simulink model "sim_Test"  (R2018a)
settings: Solver=FixedStepAuto  StartTime=0.0  StopTime=WIND(end,1)  FixedStep=0.01  RelTol=1e-3
values from neighbouring files (symbols this model uses):
  a = 0.015    [pwm_calib.mat]    (also in thr2pwm.mat)
  a1 = 3.041    [pwm_calib.mat]    (also in thr2pwm.mat)
  a2 = 1.679    [pwm_calib.mat]    (also in thr2pwm.mat)
  b = 1.686    [pwm_calib.mat]    (also in thr2pwm.mat)
  b1 = 0.1529    [pwm_calib.mat]    (also in thr2pwm.mat)
  b2 = 0.252    [pwm_calib.mat]    (also in thr2pwm.mat)
  c1 = -0.9269    [pwm_calib.mat]    (also in thr2pwm.mat)
  c2 = 1.268    [pwm_calib.mat]    (also in thr2pwm.mat)
settings Model: Creator=adiravishankara  LastModifiedBy=adiravishankara
settings DataIOCC: SaveFormat=Array

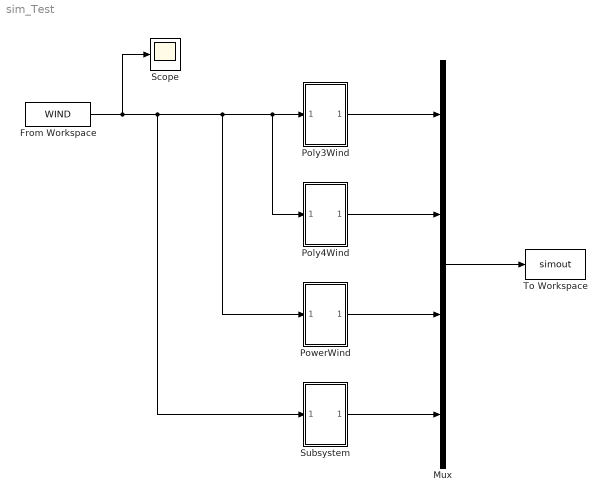
== system sim_Test ==
  From Workspace : FromWorkspace  VariableName=WIND
  Mux : Mux
  "Poly3Wind " : Subsystem
  "Poly4Wind " : Subsystem
  PowerWind : Subsystem
  Scope : Scope
  Subsystem : Subsystem
  To Workspace : ToWorkspace  VariableName=simout  SampleTime=-1
  wires:
  From Workspace/1 -> Scope/1, Subsystem/1(In1), PowerWind/1(In1), "Poly4Wind "/1(In1), "Poly3Wind "/1(In1)
  "Poly3Wind "/1(Out1) -> Mux/1
  "Poly4Wind "/1(Out1) -> Mux/2
  Subsystem/1(Out1) -> Mux/4
  PowerWind/1(Out1) -> Mux/3
  Mux/1 -> To Workspace/1

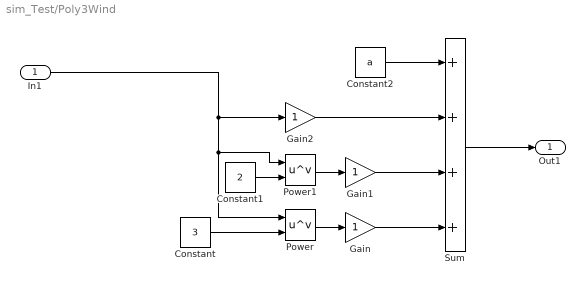
== system sim_Test/Poly3Wind  ==
  In1 : Inport
  Constant : Constant  Value=3
  Constant1 : Constant  Value=2
  Constant2 : Constant  Value=a
  Gain : Gain
  Gain1 : Gain
  Gain2 : Gain
  Power : Math  Operator=pow  SaturateOnIntegerOverflow=on
  Power1 : Math  Operator=pow  SaturateOnIntegerOverflow=on
  Sum : Sum  Inputs=++++
  Out1 : Outport
  wires:
  Constant2/1 -> Sum/1
  Constant1/1 -> Power1/2
  Gain2/1 -> Sum/2
  Sum/1 -> Out1/1
  Constant/1 -> Power/2
  Gain1/1 -> Sum/3
  In1/1 -> Gain2/1, Power1/1, Power/1
  Power1/1 -> Gain1/1
  Power/1 -> Gain/1
  Gain/1 -> Sum/4

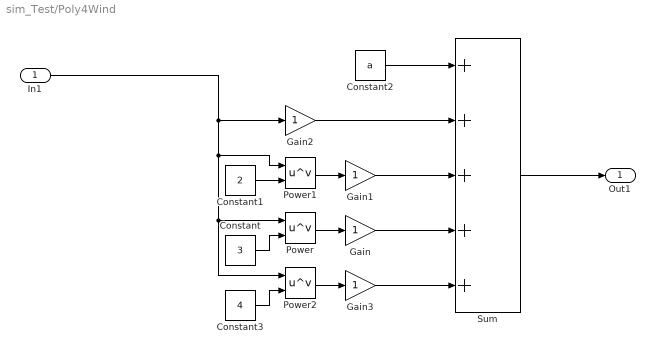
== system sim_Test/Poly4Wind  ==
  In1 : Inport
  Constant : Constant  Value=3
  Constant1 : Constant  Value=2
  Constant2 : Constant  Value=a
  Constant3 : Constant  Value=4
  Gain{,1..3} (4 alike) : Gain
  Power : Math  Operator=pow  SaturateOnIntegerOverflow=on
  Power1 : Math  Operator=pow  SaturateOnIntegerOverflow=on
  Power2 : Math  Operator=pow  SaturateOnIntegerOverflow=on
  Sum : Sum  Inputs=+++++
  Out1 : Outport
  wires:
  Gain/1 -> Sum/4
  Power/1 -> Gain/1
  Power1/1 -> Gain1/1
  In1/1 -> Power2/1, Power/1, Power1/1, Gain2/1
  Gain1/1 -> Sum/3
  Constant/1 -> Power/2
  Sum/1 -> Out1/1
  Gain2/1 -> Sum/2
  Constant1/1 -> Power1/2
  Constant2/1 -> Sum/1
  Constant3/1 -> Power2/2
  Power2/1 -> Gain3/1
  Gain3/1 -> Sum/5

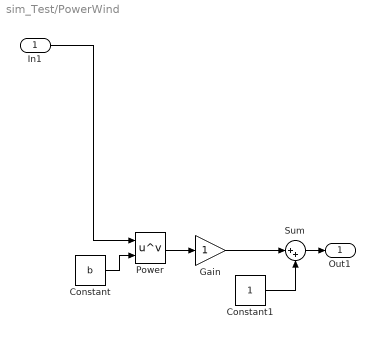
== system sim_Test/PowerWind ==
  In1 : Inport
  Constant : Constant  Value=b
  Constant1 : Constant
  Gain : Gain
  Power : Math  Operator=pow  SaturateOnIntegerOverflow=on
  Sum : Sum  Inputs=|++
  Out1 : Outport
  wires:
  Constant/1 -> Power/2
  Gain/1 -> Sum/1
  Sum/1 -> Out1/1
  In1/1 -> Power/1
  Power/1 -> Gain/1
  Constant1/1 -> Sum/2

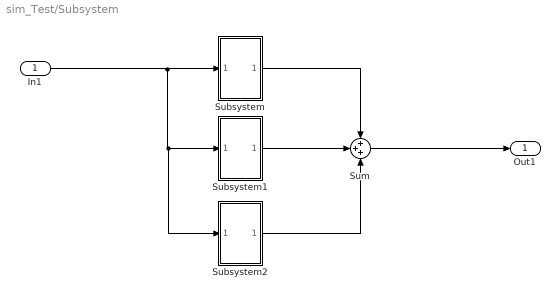
== system sim_Test/Subsystem ==
  In1 : Inport
  Subsystem : Subsystem
  Subsystem1 : Subsystem
  Subsystem2 : Subsystem
  Sum : Sum  Inputs=+++
  Out1 : Outport
  wires:
  In1/1 -> Subsystem2/1(In1), Subsystem1/1(In1), Subsystem/1(In1)
  Subsystem2/1(Out1) -> Sum/3
  Subsystem1/1(Out1) -> Sum/2
  Subsystem/1(Out1) -> Sum/1
  Sum/1 -> Out1/1

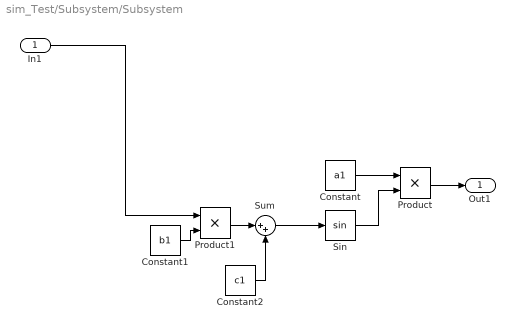
== system sim_Test/Subsystem/Subsystem ==
  In1 : Inport
  Constant : Constant  Value=a1
  Constant1 : Constant  Value=b1
  Constant2 : Constant  Value=c1
  Product : Product
  Product1 : Product
  Sin : Trigonometry
  Sum : Sum  Inputs=|++
  Out1 : Outport
  wires:
  Sin/1 -> Product/2
  Constant/1 -> Product/1
  Product1/1 -> Sum/1
  Sum/1 -> Sin/1
  Product/1 -> Out1/1
  Constant1/1 -> Product1/2
  Constant2/1 -> Sum/2
  In1/1 -> Product1/1

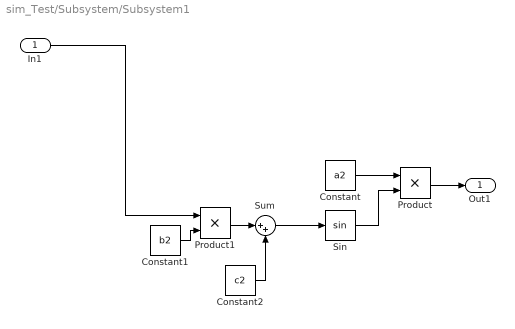
== system sim_Test/Subsystem/Subsystem1 ==
  In1 : Inport
  Constant : Constant  Value=a2
  Constant1 : Constant  Value=b2
  Constant2 : Constant  Value=c2
  Product : Product
  Product1 : Product
  Sin : Trigonometry
  Sum : Sum  Inputs=|++
  Out1 : Outport
  wires:
  In1/1 -> Product1/1
  Constant2/1 -> Sum/2
  Constant1/1 -> Product1/2
  Product/1 -> Out1/1
  Sum/1 -> Sin/1
  Product1/1 -> Sum/1
  Constant/1 -> Product/1
  Sin/1 -> Product/2

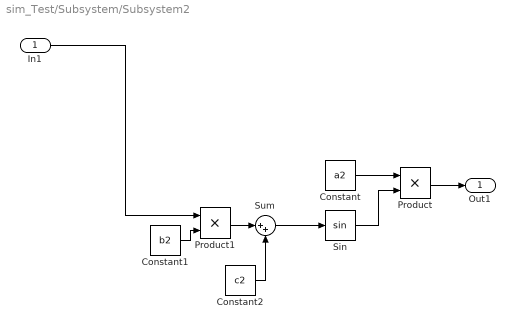
== system sim_Test/Subsystem/Subsystem2 ==
  In1 : Inport
  Constant : Constant  Value=a2
  Constant1 : Constant  Value=b2
  Constant2 : Constant  Value=c2
  Product : Product
  Product1 : Product
  Sin : Trigonometry
  Sum : Sum  Inputs=|++
  Out1 : Outport
  wires:
  Sin/1 -> Product/2
  Constant/1 -> Product/1
  Product1/1 -> Sum/1
  Sum/1 -> Sin/1
  Product/1 -> Out1/1
  Constant1/1 -> Product1/2
  Constant2/1 -> Sum/2
  In1/1 -> Product1/1
